simulink model "Kugle_sys6_block"  (R2018b)
settings: Solver=FixedStepAuto  StartTime=0.0  StopTime=10  FixedStep=0.1  RelTol=1e-3
libraries: mpclib x1, vrlib x1, simulink x1
settings Model: Creator=martinandersen  LastModifiedBy=martinandersen

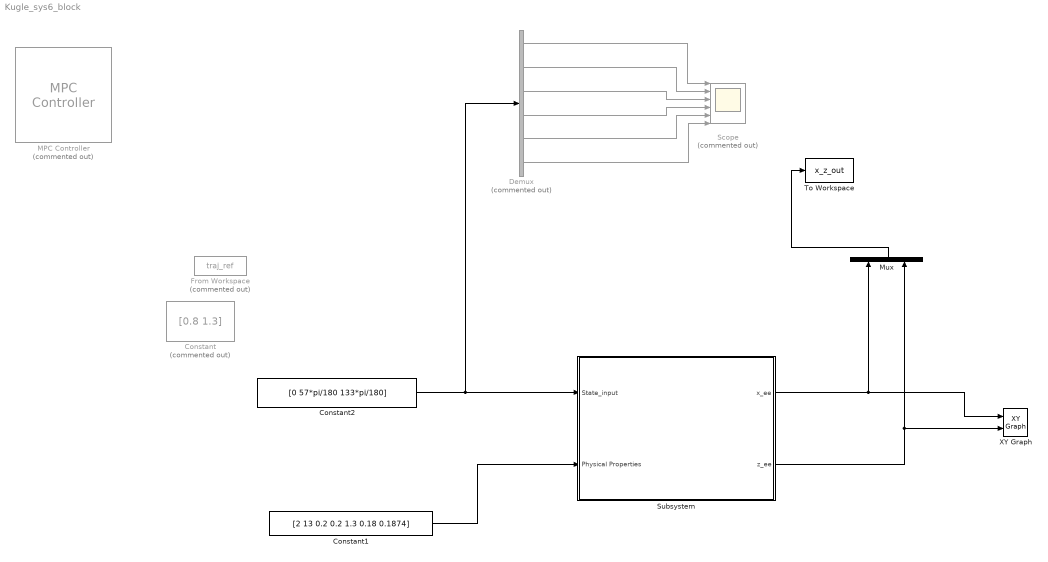
== system Kugle_sys6_block ==
  Constant : Constant  Commented=on  Value=[0.8 1.3]
  Constant1 : Constant  Value=[2 13 0.2 0.2 1.3 0.18 0.1874]
  Constant2 : Constant  Value=[0 57*pi/180 133*pi/180]
  Demux : Demux  Commented=on  Outputs=6
  From Workspace : FromWorkspace  Commented=on  VariableName=traj_ref  OutDataTypeStr=double
  MPC Controller : mpclib/MPC Controller  Commented=on  SCDEnableBlockLinearizationSpecification=on  is_multiple=0  enable_value=0  return_u0=off  updateMPCinCallerWorkspace=on  md_inport=off  mv_inport=off  return_cost=off  return_mvseq=off  return_qpstatus=off  return_xseq=off  return_state=off  return_ovseq=off  state_inport=off  umin_inport=off  umax_inport=off  ymin_inport=off  ymax_inport=off  cc_inport=off  ywt_inport=off  uwt_inport=off  duwt_inport=off  rhoeps_inport=off  uref_inport=off  n_ts=0.1  n_p=10  n_mv=3  n_md=0  n_ud=0  n_mo=2  n_uo=0  BlockDataType=double  SampleTimeInherited=off  switch_inport=off
  Mux : Mux  Inputs=2
  Scope : Scope  Commented=on  NumInputPorts=6
  Subsystem : Subsystem
  To Workspace : ToWorkspace  VariableName=x_z_out  SampleTime=-1
  XY Graph : simulink/Sinks/XY Graph  xmin=-10  xmax=10  ymin=0  ymax=2  st=-1
  wires:
  Subsystem/1(x_ee) -> XY Graph/1, Mux/1
  Subsystem/2(z_ee) -> Mux/2, XY Graph/2
  Mux/1 -> To Workspace/1
  Constant1/1 -> Subsystem/2(Physical Properties)
  Constant2/1 -> Demux/1, Subsystem/1(State_input)
  Demux/1 -> Scope/1
  Demux/2 -> Scope/2
  Demux/3 -> Scope/3
  Demux/5 -> Scope/5
  Demux/6 -> Scope/6
  Demux/4 -> Scope/4

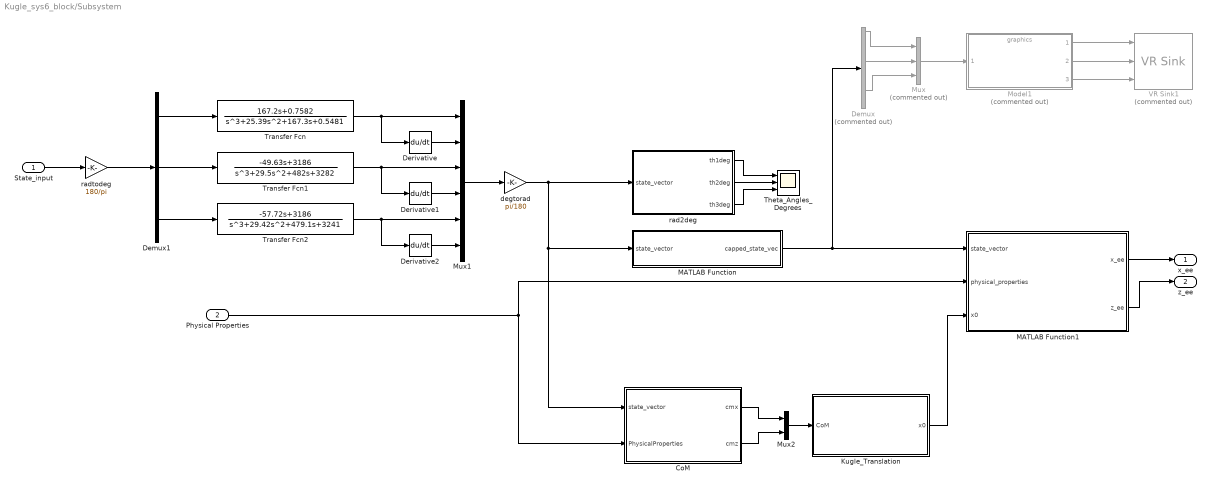
== system Kugle_sys6_block/Subsystem ==
  State_input : Inport
  Physical Properties : Inport  Port=2
  CoM : MATLAB Function  TreatAsAtomicUnit=on
  Demux : Demux  Commented=on  Outputs=6
  Demux1 : Demux  Outputs=3
  Derivative : Derivative
  Derivative1 : Derivative
  Derivative2 : Derivative
  Kugle_Translation : Subsystem
  MATLAB Function : MATLAB Function  TreatAsAtomicUnit=on
  MATLAB Function1 : MATLAB Function  TreatAsAtomicUnit=on
  Model1 : ModelReference  Commented=on  ModelNameDialog=graphics.slx  SimulationMode=Normal  ModelReferenceVersion=1.12
  Mux : Mux  Commented=on  Inputs=3
  Mux1 : Mux  Inputs=6
  Mux2 : Mux  Inputs=2
  Theta_Angles_Degrees : Scope  NumInputPorts=3
  Transfer Fcn : TransferFcn  Numerator=[167.2 0.7582]  Denominator=[1 25.39 167.3 0.5481]
  Transfer Fcn1 : TransferFcn  Numerator=[-49.63 3186]  Denominator=[1 29.5 482 3282]
  Transfer Fcn2 : TransferFcn  Numerator=[-57.72 3186]  Denominator=[1 29.42 479.1 3241]
  VR Sink1 : vrlib/VR Sink  Commented=on  InstantiateOnLoad=on  SampleTime=0.1  ViewEnable=on  RemoteChange=off  RemoteView=off  FieldsWritten=JOINT_1.rotation.4.1.1.double#JOINT_2.rotation.4.1.1.double#JOINT_3.rotation.4.1.1.double  WorldFileName=Pendel3D0.wrl  AutoView=off  VideoDimensions=[]  AllowVariableSize=off
      settings: SourceProductBaseCode=VR
  degtorad : Gain  Gain=pi/180
  rad2deg : MATLAB Function  TreatAsAtomicUnit=on
  radtodeg : Gain  Gain=180/pi
  x_ee : Outport
  z_ee : Outport  Port=2
  wires:
  MATLAB Function1/2(z_ee) -> z_ee/1
  MATLAB Function1/1(x_ee) -> x_ee/1
  Physical Properties/1 -> MATLAB Function1/2(physical_properties), CoM/2(PhysicalProperties)
  rad2deg/1(th1deg) -> Theta_Angles_Degrees/1
  rad2deg/2(th2deg) -> Theta_Angles_Degrees/2
  rad2deg/3(th3deg) -> Theta_Angles_Degrees/3
  Kugle_Translation/1(x0) -> MATLAB Function1/3(x0)
  Mux2/1 -> Kugle_Translation/1(CoM)
  CoM/1(cmx) -> Mux2/1
  CoM/2(cmz) -> Mux2/2
  MATLAB Function/1(capped_state_vec) -> Demux/1, MATLAB Function1/1(state_vector)
  State_input/1 -> radtodeg/1
  Demux1/1 -> Transfer Fcn/1
  Demux1/2 -> Transfer Fcn1/1
  Demux1/3 -> Transfer Fcn2/1
  Derivative/1 -> Mux1/2
  Derivative1/1 -> Mux1/4
  Derivative2/1 -> Mux1/6
  Mux1/1 -> degtorad/1
  Transfer Fcn/1 -> Derivative/1, Mux1/1
  Transfer Fcn1/1 -> Derivative1/1, Mux1/3
  Transfer Fcn2/1 -> Derivative2/1, Mux1/5
  Model1/1 -> VR Sink1/1
  Model1/2 -> VR Sink1/2
  Model1/3 -> VR Sink1/3
  Demux/1 -> Mux/1
  Demux/3 -> Mux/2
  Demux/5 -> Mux/3
  Mux/1 -> Model1/1
  radtodeg/1 -> Demux1/1
  degtorad/1 -> MATLAB Function/1(state_vector), CoM/1(state_vector), rad2deg/1(state_vector)

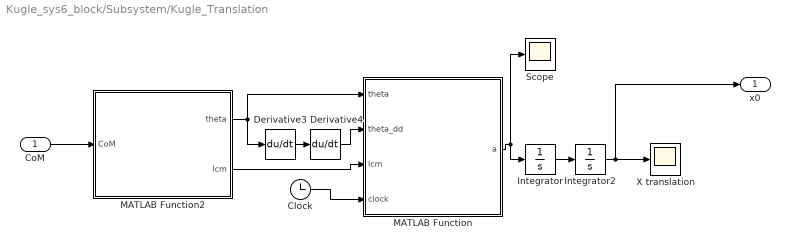
== system Kugle_sys6_block/Subsystem/Kugle_Translation ==
  CoM : Inport
  Clock : Clock
  Derivative3 : Derivative
  Derivative4 : Derivative
  Integrator : Integrator
  Integrator2 : Integrator
  MATLAB Function : MATLAB Function  TreatAsAtomicUnit=on
  MATLAB Function2 : MATLAB Function  TreatAsAtomicUnit=on
  Scope : Scope
  X translation : Scope
  x0 : Outport
  wires:
  Clock/1 -> MATLAB Function/4(clock)
  MATLAB Function/1(a) -> Integrator/1, Scope/1
  Integrator/1 -> Integrator2/1
  CoM/1 -> MATLAB Function2/1(CoM)
  MATLAB Function2/1(theta) -> Derivative3/1, MATLAB Function/1(theta)
  Derivative3/1 -> Derivative4/1
  Integrator2/1 -> x0/1, X translation/1
  Derivative4/1 -> MATLAB Function/2(theta_dd)
  MATLAB Function2/2(lcm) -> MATLAB Function/3(lcm)

== matlab function Kugle_sys6_block/Subsystem/MATLAB Function1 ==
  data: state_vector input; x_ee output; z_ee output; physical_properties input; x0 input
function [x_ee, z_ee] = fcn(state_vector, physical_properties, x0)

% Definitions
th1     = state_vector(1);
th1_d   = state_vector(2);
th2     = state_vector(3);
th2_d   = state_vector(4);
th3     = state_vector(5);
th3_d   = state_vector(6);


m0      = physical_properties(1);
m1      = physical_properties(2);
m2      = physical_properties(3);
m3      = physical_properties(4);

l1      = physical_properties(5);
l2      = physical_properties(6);
l3      = physical_properties(7);

% Velocities and accelerations


% Joint positions
T_0_1 = [cos(pi/2-th1)  -sin(pi/2-th1)  0   x0;
         sin(pi/2-th1)   cos(pi/2-th1)  0   0;
              0                0        1   0;
              0                0        0   1];
          
T_1_2 = [cos(th2)  -sin(th2)  0   l1;
         sin(th2)   cos(th2)  0   0;
             0          0     1   0;
             0          0     0   1];
         
T_2_3 = [cos(th3)  -sin(th3)  0   l2;
         sin(th3)   cos(th3)  0   0;
             0          0     1   0;
             0          0     0   1];
         
T_3_4 = [1  0  0  l3;
         0  1  0  0;
         0  0  1  0;
         0  0  0  1];
     
T_combined = T_0_1  *  T_1_2  *  T_2_3  *  T_3_4;

x_ee = T_combined(1,4);
z_ee = T_combined(2,4);

== matlab function Kugle_sys6_block/Subsystem/rad2deg ==
  data: state_vector input; th1deg output; th2deg output; th3deg output
function [th1deg, th2deg, th3deg] = fcn(state_vector)

th1deg = rad2deg(state_vector(1));
th2deg = rad2deg(state_vector(3));
th3deg = rad2deg(state_vector(5));

== matlab function Kugle_sys6_block/Subsystem/Kugle_Translation/MATLAB Function ==
  data: theta input; theta_dd input; lcm input; clock input; a output
function a = acceleration(theta, theta_dd, lcm, clock)

g = 9.81;

if clock > 0.001
    a = (lcm*theta_dd - g*sin(-theta)) / cos(-theta);
    
else
    a = 0;
end

% g = 9.81;
% 
% if clock > 0.1
%     a = (lcm*theta_dd)/(theta_d*sin(theta)) + x_d * theta_d - g;
%     
% else
%     a = 0;
% end

== matlab function Kugle_sys6_block/Subsystem/Kugle_Translation/MATLAB Function2 ==
  data: CoM input; theta output; lcm output
function [theta, lcm] = fcn(CoM)
cmx = CoM(1);
cmz = CoM(2);

%Theta1 = state_vector(1);
%Theta2 = state_vector(3);
%Theta3 = state_vector(5);

%[cmx, cmz] = CMcalculator(Theta1, Theta2, Theta3, PhysicalProperties);

lcm = sqrt(cmx^2 + cmz^2);


theta = sign(cmx)*acos(cmz/lcm);

== matlab function Kugle_sys6_block/Subsystem/CoM ==
  data: state_vector input; cmx output; PhysicalProperties input; cmz output
function [cmx, cmz] = CoM(state_vector, PhysicalProperties)
Theta1 = state_vector(1);
Theta2 = state_vector(3);
Theta3 = state_vector(5);

[cmx, cmz] = CMcalculator(Theta1, Theta2, Theta3, PhysicalProperties);

== matlab function Kugle_sys6_block/Subsystem/MATLAB Function ==
  data: state_vector input; capped_state_vec output
function capped_state_vec = fcn(state_vector)

capped_state_vec = state_vector;

if(state_vector(3) > deg2rad(100))
    capped_state_vec(3) = deg2rad(100);
    
elseif (state_vector(3) < deg2rad(-57))
    capped_state_vec(3) = deg2rad(-57);

end
    
if (state_vector(5) > deg2rad(133))
    capped_state_vec(5) = deg2rad(133);
    
elseif(state_vector(5) < 90-deg2rad(state_vector(3)))
    capped_state_vec(5) = 90-deg2rad(state_vector(3));
    
end
